simulink library "carnot"  (R2013b)
settings: Solver=ode45  StartTime=0.0  StopTime=10.0  RelTol=1e-3
undefined symbols (not defined in the file or in its folder): A, acol, Ahabit, Awin, Azimuth_Angle, AziWin, B, C, c1, c4, capc, caph, CarnotCallbacks_Density, CarnotCallbacks_Enthalpy, CarnotCallbacks_Enthalpy2Temperature, CarnotCallbacks_Entropy, CarnotCallbacks_Evaporation_Enthalpy, CarnotCallbacks_GlobalMessageLevel, CarnotCallbacks_Grashof, CarnotCallbacks_Heat_Capacity, CarnotCallbacks_Kinematic_Viscosity, CarnotCallbacks_Prandtl, CarnotCallbacks_Saturation_Property, CarnotCallbacks_Saturation_Temperature, CarnotCallbacks_Saturation_Value_Water, CarnotCallbacks_Specific_Volume, CarnotCallbacks_Thermal_Conductivity, CarnotCallbacks_Vapour_Content, CarnotCallbacks_Vapour_Pressure, con, cond, d, Dd, density, dfin, dia, DiameterLastPiece, DPConstant, dpipe, DPLinear, DPQuadratic, emission_out, fluid, FluidMix, FluidType, FPC, frame, g, GeodeticHeight, Gwin, heat_capacity, hgt, HP, Hroom, ID, inlet, K, l, lin, lpipe ... (+29)
undefined symbols (not defined in the file): c2, c3, c5, c6, cwall, dactive, height, mc, mID, rho, tau, UAneighbour, UAwall, uloss
libraries: carnot x333, simulink x25, simulink_extras x7
(part 6 of 16)

== system carnot/Load/Hot_Water_Tapping ==
  Applications : Subsystem
      mask Display: plot(0,0,100,100,[10,10,40,40,10],[10,40,40,10,10],[50,70,90,50],[30,65,30,30],[20,10,10,20,30,40,40,30,20],[50,60,70,80,80,70,60,50,50])
  DHW_Energy_Tapping : Subsystem  mask{mdot_nom=1/60, times=[7     7.1 7.5   8.083 8.25  8.5   8.75  9     9.5   10.5  11.5  11.75 12.75 14.5  15.5  16.5  18    18.25 18.5  19    20.5  21.25 21.5]*3600, energies=[0.105 1.4 0.105 0.105 0.105 0.105 0.105 0.105 0.105 0.105 0.105 0.105 0.315 0.105 0.105 0.105 0.105 0.105 0.105 0.105 0.735 0.105 1.4 ]*36e5, dT_set=[30    30  30    30    30    30    30    30    30    30    30    30    45    30    30    30    30    30    30    30    45    30    30  ], coeffs=[3     6   3     3     3     3     3     3     3     3     3     3     4     3     3     3     3     3     3     3     4     3     6   ]}
      mask prompts: mdot_nom "nominal massflow [kg/s]"; times "vector of start times of taps [s]"; energies "vector of energies of taps [J]"; dT_set "vector of delta set temperatures of taps [K]"; coeffs "vector of coefficients of nominal massflow of taps [-]"
      mask Display: disp('dhw_EN13203')
  EU_Tapping_Cycle : Subsystem  mask(European tapping cycles){eu_tap=L}
      mask prompts: eu_tap "EU Tapping Cycle Number"
      mask help: European tapping cycles according to EN 13203.
      mask init:
      | % times in h, energies in kWh, massflow in kg/min
      | % will be transformed to s, J at kg/s the end
      | switch(eu_tap)
      |     case 1  % profile 3XS   0.345 kWh
      |         times =    [7.000   7.083   7.250   7.433   7.500   9.000   9.500   11.50   11.75   12.00   12.50   12.75   14.50   15.00   15.50   16.00   18.50   19.00   19.50   21.25   21.50   21.58   21.75 ];
      |         energies = [0.015   0.015   0.015   0.015   0.015   0.015   0.015   0.015   0.015   0.015   0.015   0.015   0.015   0.015   0.015   0.015   0.015   0.015   0.015   0.015   0.015   0.015   0.015 ];
      |         dT_set =   [30      30      30      30      30      30      30      30      30      30      30      30      30      30      30      30      30      30      30      30      30      30      30  ];
      |         mdot =     [2       2       2       2       2       2       2       2       2       2       2       2       2       2       2       2       2       2       2       2       2       2       2   ];
      | 
      |     case 2  % profile XXS   2.1 kWh
      |         times =    [7.000   7.500   8.500   9.500   11.50   11.75   12.00   12.50   12.75   18.00   18.25   18.50   19.00   19.50   20.00   20.75   21.00   21.25   21.58   21.75 ];
      |         energies = [0.105   0.105   0.105   0.105   0.105   0.105   0.105   0.105   0.105   0.105   0.105   0.105   0.105   0.105   0.105   0.105   0.105   0.105   0.105   0.105 ];
      |         dT_set =   [30      30      30      30      30      30      30      30      30      30      30      30      30      30      30      30      30      30      30      30    ];
      |         mdot =     [2       2       2       2       2       2       2       2       2       2       2       2       2       2       2       2       2       2       2       2     ];
      | 
      |     case 3  % profile XS    2.1 kWh
      |         times =    [7.500   12.75   21.50   ];
      |         energies = [0.525   0.525   1.05    ];
      |         dT_set =   [30      30      30      ];
      |         mdot =     [3       3       3       ];
      |     
      |     case 4  % profile S     2.1 kWh
      |         times =    [7.000   7.500   8.500   9.500   11.50   11.75   12.75   18.00   18.25   20.50   21.50   ];
      |         energies = [0.105   0.105   0.105   0.105   0.105   0.105   0.315   0.105   0.105   0.420   0.525   ];
      |         dT_set =   [30      30      30      30      30      30      45      30      30      45      30      ];
      |         mdot =     [3       3       3       3       3       3       4       3       3       4       5       ];
      |     
      |     case 5 % Profile M      5.845 kWh
      |         times =    [7.000 7.083 7.500 8.016 8.250 8.5   8.750 9.000 9.500 10.50 11.50 11.75 12.75 14.50 15.50 16.50 18.00 18.25 18.50 19.00 20.50 21.25 21.5];
      |         energies = [0.105 1.4   0.105 0.105 0.105 0.105 0.105 0.105 0.105 0.105 0.105 0.105 0.315 0.105 0.105 0.105 0.105 0.105 0.105 0.105 0.735 0.105 1.4 ];
      |         dT_set =   [30    30    30    30    30    30    30    30    30    30    30    30    45    30    30    30    30    30    30    30    45    30    30  ];
      |         mdot   =   [3     6     3     3     3     3     3     3     3     3     3     3     4     3     3     3     3     3     3     3     4     3     6   ];
      |         
      |     case 6 % profile L      11.655 kWh
      |         times =    [7.000 7.083 7.500 7.750 8.083 8.416 8.500 8.750 9.000 9.500 10.50 11.50 11.75 12.75 14.50 15.50 16.50 18.00 18.25 18.50 19.00 20.50 21.00 21.5 ];
      |         energies = [0.105 1.4   0.105 0.105 3.605 0.105 0.105 0.105 0.105 0.105 0.105 0.105 0.105 0.315 0.105 0.105 0.105 0.105 0.105 0.105 0.105 0.735 3.605 0.105];
      |         dT_set   = [30    30    30    30    30    30    30    30    30    30    30    30    30    45    30    30    30    30    30    30    30    45    30    30   ];
      |         mdot     = [3     6     3     3     10    3     3     3     3     3     3     3     3     4     3     3     3     3     3     3     3     4     10    3    ];
      |         
      |     case 7  % profile XL      19.07 kWh
      |         times =    [7.000 7.25  7.433 7.75  8.016 8.250 8.500 8.750 9.000 9.500 10.00 10.50 11.00 11.50 11.75 12.75 14.50 15.00 15.50 16.00 16.50 17.00 18.00 18.25 18.50 19.00 20.50 20.76 21.25 21.5 ];
      |         energies = [0.105 1.82  0.105 4.42  0.105 0.105 0.105 0.105 0.105 0.105 0.105 0.105 0.105 0.105 0.105 0.735 0.105 0.105 0.105 0.105 0.105 0.105 0.105 0.105 0.105 0.105 0.735 4.420 0.105 4.42 ];
      |         dT_set   = [30    35    30    30    30    30    30    30    30    30    30    30    30    30    45    45    30    30    30    30    30    30    30    35    35    30    45    35    30    35   ];
      |         mdot     = [3     6     3     10    3     3     3     3     3     3     3     3     3     4     3     3     3     3     3     3     3     4     10    3     3     3     4     10    3     10   ];
      |         
      |     case 8  % profile XXL      24.53 kWh
      |         times =    [7.000 7.25  7.433 7.75  8.016 8.250 8.500 8.750 9.000 9.500 10.00 10.50 11.00 11.50 11.75 12.75 14.50 15.00 15.50 16.00 16.50 17.00 18.00 18.25 18.50 19.00 20.50 20.76 21.25 21.5 ];
      |         energies = [0.105 1.82  0.105 6.24  0.105 0.105 0.105 0.105 0.105 0.105 0.105 0.105 0.105 0.105 0.105 0.735 0.105 0.105 0.105 0.105 0.105 0.105 0.105 0.105 0.105 0.105 0.735 6.240 0.105 6.24 ];
      |         dT_set   = [30    35    30    35    30    30    30    30    30    30    30    35    30    45    45    45    30    30    30    30    30    30    30    35    35    30    45    35    35    35   ];
      |         mdot     = [3     6     3     10    3     3     3     3     3     3     3     3     4     3     3     4     3     3     3     3     3     3     3     3     3     3     4     16    10    16   ];
      |         
      |     case 9  % profile 3XL      46.76 kWh
      |         times =    [7.00  8.016 9.000 10.50 11.75 12.75 15.50 18.50 20.50 21.5 ];
      |         energies = [11.2  5.04  1.68  0.840 1.68  2.520 2.520 3.36  5.88  12.04];
      |         dT_set   = [35    30    30    35    30    45    30    30    45    35   ];
      |         mdot     = [48    24    24    24    24    32    24    24    32    48   ];
      |         
      |     case 10 % profile 4XL      93.52 kWh
      |         times =    [7.000 8.016 9.000 10.50 11.75 12.75 15.50 18.50 20.50 21.5 ];
      |         energies = [22.40 10.08 3.36  1.680 3.360 5.04  5.04  6.72  11.76 24.08];
      |         dT_set   = [35    30    30    30    30    45    30    30    45    35   ];
      |         mdot     = [96    48    48    10    48    64    48    48    64    96   ];
      |         
      |     otherwise
      |         disp('Wrong definition of tapping profile')
      | end
      | energies = energies*36e5;
      | times = times*3600;
      | mdot = mdot/60;
      mask TypeOptions eu_tap: 3XS | XXS | XS | S | M | L | XL | XXL | 3XL | 4XL
      mask Display: disp('EU tapping\n from 3XS\nto 4XL')
  T_cold_Water_Location : Subsystem  mask(water tap){loc=Wuerzburg}
      mask prompts: loc "Location"
      mask help:
      | The block models a tap, that produces a constant massflow of a fluid at given times.
      | control = 1 is full massflow, control = 0 is no massflow.
      | The temperature is a sine wave according to:
      |
      | T(out) = T(mean) + T(amplitude) * sin( 2*PI*(SimulationDay + DayPhaseShift) / 365 )
      mask init:
      | switch loc
      |     case 1  % Athens
      |         T = 15;
      |         Tamp = 5;
      |         dshift = -20;
      |         disp('check temperatures for Athens')
      |     case 2  % Barcelona
      |     case 4  % Madrid
      |         T = 13.5;
      |         Tamp = 4.5;
      |         dshift = -19;
      |     case 3  % Lyon
      |         T = 12;
      |         Tamp = 4;
      |         dshift = -80;
      |         disp('check temperatures for Lyon')
      |     case 5  % Stockholm
      |         T = 8.5;
      |         Tamp = 6.4;
      |         dshift = -80;
      |         disp('check temperatures for Stockholm')
      |     case 6  % Wuerzburg
      |         T = 10;
      |         Tamp = 3;
      |         dshift = -137;
      |     case 7  % Zuerich        
      |         T = 9.7;
      |         Tamp = 6.3;
      |         dshift = -60;
      |         disp('check temperatures for Zuerich')
      |     otherwise
      |         T = 10;
      |         Tamp = 3;
      |         dshift = -137;
      | end
      mask Help: eval('man (''water_tap'')')
      mask TypeOptions loc: Athens | Barcelona | Lyon | Madrid | Stockholm | Wuerzburg | Zuerich
      mask Display:
      | str = ['Athens   ';'Barcelona';'Lyon     ';'Madrid   ';'Stockholm';'Wuerzburg';'Zuerich  '];
      | disp(str(loc,:))
  T_cold_Water_Season : Subsystem  mask(water tap){form=sine wave, month1=February, temp1=6, month2=August, temp2=14}
      mask prompts: form "temperature distribution"; month1 "month with min. temp"; temp1 "minimal temperature [°C]"; month2 "month with max. temp"; temp2 "maximal temperature [°C]"
      mask help:
      | The block models a tap, that produces a constant massflow of a fluid at given times.
      | control = 1 is full massflow, control = 0 is no massflow.
      | The temperature of the water varies during the year.
      mask Help: eval('man (''water_tap'')')
      mask TypeOptions form: sine wave | linear
      mask TypeOptions month1: January | February | March | April | May | June | July | August | September | October | November | December
      mask TypeOptions month2: January | February | March | April | May | June | July | August | September | October | November | December
      mask Display: plot(0,-10,115,110,[0,0],[100,0],[100,0],[50,50],[100,70,20,0],[44,70,30,44])
  T_cold_Water_Sine : Subsystem  mask(water tap){T=10, Tamp=3, dshift=-137}
      mask prompts: T "mean temperature [degree centigrade]"; Tamp "amplitude of the sine [k]"; dshift "phase shift of the sine in [days]"
      mask help:
      | The block models a tap, that produces a constant massflow of a fluid at given times.
      | control = 1 is full massflow, control = 0 is no massflow.
      | The temperature is a sine wave according to:
      |
      | T(out) = T(mean) + T(amplitude) * sin( 2*PI*(SimulationDay + DayPhaseShift) / 365 )
      mask Help: eval('man (''water_tap'')')
      mask Display: plot(0,-10,115,110,[0,0],[100,0],[100,0],[50,50],[100,90,80,70,60,50,40,30,20,10,0],[50,38,30,30,38,50,61,69,69,61,50])
  Water_Tap : Subsystem  mask(water tap){dia=0.02, p=2e5}
      mask prompts: dia "diameter at outlet [m]"; p "system pressure [Pa]"
      mask help:
      | The block models a tap, that produces a constant massflow of a fluid at given times.
      | control = 1 is full massflow, control = 0 is no massflow.
      mask init:
      | fluid = 1; %water
      | mix = 0;
      | dia = max(0.001, dia);
      | p = max(p, 0);
      mask Help: eval('man (''water_tap'')')
      mask Display: plot(-10,10,90,90,[44,67,67,45,45,40,40,44],[80,80,72,72,60,60,76,80],[60,45],[90,90],[53,53],[80,90],[24,29,70,75,24],[30,10,10,30,30],[42,42],[32,58],[46,44],[34,54],[38,40],[34,56])
  create_mdot : Subsystem  mask(Create Massflow Profile){}
      settings: OpenFcn=CarnotCallbacks_create_mdot('initialize',gcb);
      mask Help: web(fullfile(path_carnot('help'),'create_mdot.html'),'-helpbrowser')
  mdot_40_20_40 : Subsystem  mask(Repeating Tapping Profile){period=24*3600, rep_seq_t=[7 12 19]*3600, rep_seq_d=[0.2 0.1 0.2]*3600, rep_seq_y=[1 1 1]*200/1800}
      mask prompts: period "Time period in s"; rep_seq_t "Time values in s"; rep_seq_d "Duration in s"; rep_seq_y "Output values:"
      mask help:
      | Period must be larger than the last time value.
      | Time values must be monotonically ingreasing. Give one time value for the start of the tapping.
      | Duration is a vector with the same number of elements than the time values. Each duration corresponts to one time value.
      | The number of output values must be the same as the number of time values. Each output value corresponds to one time value.
      mask init: same as carnot/Load/General/Repeating_Profile
      mask Help:
      | Period must be larger than the last time value.
      | Time values must be monotonically ingreasing. Give one time value for the start of the tapping.
      | Duration is a vector with the same number of elements than the time values. Each duration corresponts to one time value.
      | The number of output values must be the same as the number of time values. Each output value corresponds to one time value.
      mask Display: plot( disp_t, disp_y )
  mdot_DHWcalc : Subsystem  mask(dhw from file){file=DHW0001_DHW, ext=.txt, dt=60}
      mask prompts: file "Name of file"; ext "Extension of file"; dt "Time step duration [s]"
      mask help:
      | Input for files created with the dhw-calc software.
      | These files contain only the massflow in kg/h, the conversion to kg/s is done in the block.
      | Details and manual at
      | http://solar.umwelt-uni-kassel.de/downloads.de.html
      mask init:
      | eval(['load(''' file ext ''');']);
      | eval([file ' = [ [0:dt:(length(' file ')-1)*dt]'' ' file '];' ]);
      | set_param([gcb '/dhw_from_Workspace'], 'VariableName', file);
      mask Help: eval('man (''dhw_from_file'')')
      mask TypeOptions ext: .dat | .txt
      mask Display: disp(file)

== system carnot/Load/Houses ==
  Room_Floor_Heating : Subsystem  mask(room){t0=20, temp_neighbour=20}
      mask prompts: t0 "start temperature of rooms in °C"; temp_neighbour "temperature of rooms above and below in °C"
      mask help:
      | The block models of a heat transfer characteristic of two neighbour rooms.
      | Use "look under mask" to set up the models parameters (initial conditions,
      | floors and wall characteristics...)
      mask init:
      | AIV_neighbour = [0 temp_neighbour temp_neighbour 0 0 0 0 0 0];
      | zonefloordist2grnd = 0;
      mask Help: web(fullfile(path_carnot('help'),'Room_Floor_Heating.html'),'-helpbrowser')
      mask Display: plot(0,0,100,100,[30,30,60,60,30],[20,50,50,20,20],[47,47,56,56,47],[40,30,30,40,40],[42,42,34,34],[20,40,40,20],[62,45,28],[48,70,48])
  Room_Radiator : Subsystem  mask(room){t0=20, temp_neighbour=20}
      mask prompts: t0 "start temperature of rooms in °C"; temp_neighbour "temperature of rooms above and below in °C"
      mask help:
      | The block models of a heat transfer characteristic of two neighbour rooms.
      | Use "look under mask" to set up the models parameters (initial conditions,
      | floors and wall characteristics...)
      mask init:
      | AIV_neighbour = [0 temp_neighbour temp_neighbour 0 0 0 0 0 0];
      | zonefloordist2grnd = 0;
      mask Help: web(fullfile(path_carnot('help'),'Room_Radiator.html'),'-helpbrowser')
      mask Display: plot(0,0,100,100,[30,30,60,60,30],[20,50,50,20,20],[47,47,56,56,47],[40,30,30,40,40],[42,42,34,34],[20,40,40,20],[62,45,28],[48,70,48])
  Simple_House : Subsystem  mask(simple house){Ahabit=30, Hroom=2.5, Floorsize=[5 6], UAwall=0.162*(30)+0.182*((5+6)*2*2.5 -(4+0+0+0)), UAneighbour=0, Uground=0  %0.18 wenn Wert verlangt, mc=0.5e6*30   % 0.5 MJ/m2/K, shade=0.75, tini=20, Awin=[4 0 0 0], AziWin=[0 90 -180 -90], Uwin=[1    1   1    1]*1.5, Gwin=[1    1   1    1]*0.7*(1-0.15), vent=0.4, rec=0, heatload=2000, dpcoeff=[10 100], delta_t_nom=50, n_rad=1.1, mass_times_cap=40e6}
      mask prompts: Ahabit "Living surface in m²"; Hroom "height of rooms in m"; Floorsize "Dimensions of slab in m [length width]"; UAwall "Total heat transfer to ambient (walls/roof) in W/K"; UAneighbour "Total heat transfer to neighbour inW/K"; Uground "Heat transfer coeffient to ground in W/m²/K"; mc "Total thermal capacity in J/K"; shade "Shading factor [0..1] when T room > 4 K + T_init"; tini "Initial temperature"; Awin "Surface of 4 windows in m² (vector)"; AziWin "Orientation of 4 windows (south 0, east -90,west 90)"; Uwin "Heat loss coefficient 4 windows in W/m²/K [vector]"; Gwin "Light transmittance 4 windows (0..1) * (1 - frame_part) [vector]"; vent "Ventilation rate in 1/h"; rec "Heat recovery (0..1)"; heatload "Heating capacity radiator  [W]"; dpcoeff "Pressure drop coefficients [linear quadratic] in Pa/(kg/s), Pa/(kg/s)²"; delta_t_nom "Nominal delta T (average radiator temperature - room temperature) [K]"; n_rad "Radiator exponent"; mass_times_cap "Mass*capacity of heating system [J/K]"
      mask help:
      | Simple model of 1-node room or house. The differential equation
      | (m*c)house * dT/dt = solar_gain + internal_gain + heating_power - losses_to_ambient - losses_to_neighbour_room
      | is solved.
      | The heating power is generated by a radiator or floor heating system.
      | The windows have an automatic shading (shading factor) if room temperature rises 4 K above initial temperature.
      | solar gain = Solar_Radiation_on_window * light_transmittance * shading_factor
      | Use "look under mask" to set up the models parameters (initial conditions, surfaces characteristics...).
      | A usual value for the internal gains is 2.3 W/m².
      mask init:
      | invmc = 1/mc;
      | rec = max(0,min(1,rec));
      | Gwin = max(0,min(1,Gwin));
      | shade = max(0, min(1, shade));
      mask Help: web(fullfile(path_carnot('help'),'simple_house.html'),'-helpbrowser')
      mask Display: plot(0,-15,80,100,[30,30,60,60,30],[20,50,50,20,20],[47,47,56,56,47],[40,30,30,40,40],[42,42,34,34],[20,40,40,20],[62,45,28],[48,70,48])
  Simple_House_ISO_GroundModel : Subsystem  mask(Simple House with ISO 13370 Ground Model){Ahabit=140, Hroom=2.6, Floorsize=[7 10], UAwall=0.162*(54.6+26.4)+0.182*((45.7+56.0)*2 -(12+4+3+4)), UAneighbour=0, Uground=0.1, mc=0.5e6*140 % 0.5 MJ/m2/K, shade=0.75, tini=20, Awin=[12 4 3 4], AziWin=[0 90 -180 -90], Uwin=[1    1   1    1]*1.0, Gwin=[1    1   1    1]*0.585*(1-0.15), vent=0.4, rec=0.6, heatload=1792, delta_t_nom=15, n_rad=1.1, mass_times_cap=40e6, dpcoeff=[10 100]}
      mask prompts: Ahabit "Living surface in m²"; Hroom "height of rooms in m"; Floorsize "Dimensions of slab in m [length width]"; UAwall "Total heat transfer to ambient (walls/roof) in W/K"; UAneighbour "Total heat transfer to neighbour inW/K"; Uground "Heat transfer coeffient of slab to ground in W/m²/K"; mc "Total thermal capacity in J/K"; shade "Shading factor [0..1] when T room > 4 K + T_init"; tini "Initial temperature"; Awin "Surface of 4 windows in m² (vector)"; AziWin "Orientation of 4 windows (south 0, east -90,west 90)"; Uwin "Heat loss coefficient 4 windows in W/m²/K [vector]"; Gwin "Light transmittance 4 windows (0..1) * (1 - frame_part) [vector]"; vent "Ventilation rate in 1/h"; rec "Heat recovery (0..1)"; heatload "Heating capacity radiator  [W]"; delta_t_nom "Nominal delta T (average radiator temperature - room temperature) [K]"; n_rad "Radiator exponent"; mass_times_cap "Mass*capacity of heating system [J/K]"; dpcoeff "Pressure drop coefficients [linear quadratic] in Pa/(kg/s), Pa/(kg/s)²"
      mask help:
      | Uses the simple model of 1-node room or house. The heating power is generated by a radiator or floor heating system.
      | The windows have an automatic shading (shading factor) if room temperature rises 4 K above initial temperature.
      | solar gain = Solar_Radiation_on_window * light_transmittance * shading_factor
      | The ground model of ISO 13370 is used to calculate the losses to the ground. Remember to set the values of the model according to the set point of the room temperature and the weather data.
      mask init:
      | invmc = 1/mc;
      | rec = max(0,min(1,rec));
      | Gwin = max(0,min(1,Gwin));
      | shade = max(0, min(1, shade));
      mask Help: web(fullfile(path_carnot('help'),'simple_house.html'),'-helpbrowser')
      mask Display:
      | plot(-20,-30,120,100,[10,10,90,90,10],[0,50,50,0,0],...
      |     [100,60,40,0],[40,80,80,40],[20,34,34,20,20],[40,40,20,20,40],...
      |     [60,60,40,40],[0,40,40,0],[65,80,80,65,65],[40,40,20,20,40],...
      |     [47,54,54,47,47],[35,35,4,4,35],[45,41],[20,20])
  Simple_House_ISOgm_CONF : Subsystem  mask(Simple House with ISO 13370 Ground Model){parameterfile=Default_SimpleHouseISOgm, tini=20}
      mask prompts: parameterfile "Parameter set"; tini "Initial temperature in °C"
      mask help: Preconfigurated parameter sets.
      mask init:
      | % path definitions
      | intpath = fullfile(path_carnot('intlibsl'), ...
      |     'Load','Houses','Simple_House_ISOgm_CONF','parameter_set');
      | pubpath = fullfile(path_carnot('libsl'), ...
      |     'Load','Houses','Simple_House_ISOgm_CONF','parameter_set');
      | 
      | [namelist, lib] = CarnotCallbacks_getConfNamelist(intpath,pubpath);
      | 
      | if ~lib
      |     myMaskStylesVar{1} = ['popup(', namelist,')'];
      |     myMaskStylesVar{2} = 'edit';
      |     set_param(gcb, 'MaskStyles', myMaskStylesVar)
      | end
      | 
      | if exist(fullfile(intpath,[parameterfile '.mat']))
      |     load(fullfile(intpath,parameterfile));
      | else
      |     load(fullfile(pubpath,parameterfile));
      | end
      mask Help: web(fullfile(path_carnot('help'),'simple_house.html'),'-helpbrowser')
      mask TypeOptions parameterfile: Default_SimpleHouseISOgm
      mask Display:
      | % user defined picture file
      | picfile = fullfile(path_carnot('intlibsl'), ...
      |         'Load','Houses','Simple_House_ISOgm_CONF','parameter_set', ...
      |         'Simple_House_ISOgm_CONF.jpg');
      | 
      | % show internal picture if defined
      | if ~BlockIsInCarnotLibrary ...      % if not located in library any more
      |         && exist(picfile,'file')    % AND picfile is present
      |     image(imread(picfile), [0.15 0.1 0.7 0.8])
      |     set_param(gcb, 'BackgroundColor', 'White')
      | else
      |     % show public picture
      |     plot([10,10,90,90,10]/100,[0,50,50,0,0]/100,...
      |          [100,60,40,0]/100,[40,80,80,40]/100,...
      |          [20,34,34,20,20]/100,[40,40,20,20,40]/100,...
      |          [60,60,40,40]/100,[0,40,40,0]/100,...
      |          [65,80,80,65,65]/100,[40,40,20,20,40]/100,...
      |          [47,54,54,47,47]/100,[35,35,4,4,35]/100,...
      |          [45,41]/100,[20,20]/100)
      |     set_param(gcb, 'BackgroundColor', 'Orange')
      | end
      | 
      | % port labels
      | port_label('input',1,'WDB')
      | port_label('input',2,'THB')
      | port_label('output',1,'Hdat')
      | port_label('output',2,'THB')
  heat_transfer : Subsystem
      mask Display: plot(0,0,100,100,[10,10,40,40,10],[10,40,40,10,10],[50,70,90,50],[30,65,30,30],[20,10,10,20,30,40,40,30,20],[50,60,70,80,80,70,60,50,50])
  room_nodes : Subsystem
      mask Display: plot(0,0,100,100,[10,10,40,40,10],[10,40,40,10,10],[50,70,90,50],[30,65,30,30],[20,10,10,20,30,40,40,30,20],[50,60,70,80,80,70,60,50,50])
  ventilation_heating : Subsystem
      mask Display: plot(0,0,100,100,[10,10,40,40,10],[10,40,40,10,10],[50,70,90,50],[30,65,30,30],[20,10,10,20,30,40,40,30,20],[50,60,70,80,80,70,60,50,50])
  wall_floor : Subsystem
      mask Display: plot(0,0,100,100,[10,10,40,40,10],[10,40,40,10,10],[50,70,90,50],[30,65,30,30],[20,10,10,20,30,40,40,30,20],[50,60,70,80,80,70,60,50,50])

== system carnot/New_Blocks/ReadFile ==
  S-Function : S-Function  FunctionName=readfile  Parameters=number timedep filename  EnableBusSupport=off
  dummy constant : Constant  Value=0
  data : Outport
  wires:
  dummy constant/1 -> S-Function/1
  S-Function/1 -> data/1

== system carnot/New_Blocks/ground_storage_U_tube ==
  WDB : Inport
  THBin : Inport  Port=2
  Tsurface : Inport  Port=3
  Tbottom : Inport  Port=4
  Demux : Demux  Outputs=[3*mpts 1 1 3]
  Demux1 : Demux  Outputs=[1 1 1 1 2 1 3]
  Demux2 : Demux  Outputs=[10 10]
  Matrix Gain : Gain  Gain=[1-1/zn:-1/zn:0]'  SaturateOnIntegerOverflow=on  OutDataTypeStr=Inherit: Same as input  ParamDataTypeStr=Inherit: Same as input
  Mux : Mux  Inputs=10
  Mux1 : Mux  Inputs=8
  Open_Surface : carnot/Storage/Thermal/surface_models/Open_Surface  albedo=0.6
  S-Function : S-Function  FunctionName=ut_stor2  Parameters=ds, hs, ce, le, dp, dh, hh, ch, lh, kp, t0, rn, zn, mpts  EnableBusSupport=off
  Sum : Sum  Inputs=+-  SaturateOnIntegerOverflow=on  InputSameDT=on  OutDataTypeStr=Inherit: Same as first input
  Sum1 : Sum  SaturateOnIntegerOverflow=on  InputSameDT=on  OutDataTypeStr=Inherit: Same as first input
  THB2THV : carnot/Toolbox/THB2THV
  THV2THB : carnot/Toolbox/THV2THB
  diameter : Constant  Value=dp
  THB : Outport
  Tnodes : Outport  Port=2
  wires:
  Mux1/1 -> THV2THB/1
  Demux/1 -> Tnodes/1
  Demux/4 -> Mux1/7  "clq"
  Demux1/7 -> Mux/8  "clq"
  Sum1/1 -> Mux/9
  Demux/2 -> Mux1/2  "Tout"
  Demux/3 -> Mux1/4  "p_out"
  S-Function/1 -> Demux/1
  WDB/1 -> Open_Surface/1
  diameter/1 -> Mux1/6
  Demux2/2 -> Mux1/8
  THBin/1 -> THB2THV/1
  Demux2/1 -> Demux1/1
  Open_Surface/1 -> Mux/1
  Demux1/1 -> Mux/2, Mux1/1  "ID"
  Mux/1 -> S-Function/1
  Demux1/2 -> Mux/3  "T"
  Demux1/4 -> Mux/5  "p"
  Demux1/6 -> Mux/7  "d"
  Demux1/3 -> Mux/4, Mux1/3  "mdot"
  Demux1/5 -> Mux/6, Mux1/5  "fluid, mix"
  Tsurface/1 -> Sum/1
  Sum/1 -> Matrix Gain/1
  Matrix Gain/1 -> Sum1/1
  Tbottom/1 -> Sum/2, Mux/10, Sum1/2
  THB2THV/1 -> Demux2/1
  THV2THB/1 -> THB/1

== system carnot/Outputs/AIV_selector ==
  "[AIV]" : Inport
  Selector : Selector  InputPortWidth=9  IndexOptions=Index vector (dialog)  Indices=v  OutputSizes=1
  "[AIV]s" : Outport
  wires:
  Selector/1 -> "[AIV]s"/1
  "[AIV]"/1 -> Selector/1

== system carnot/Outputs/Display_THB1 ==
  THB_yellow : Inport
  Selector : Selector  InputPortWidth=20  IndexOptions=Index vector (dialog)  Indices=[v]  OutputSizes=1
  THB2THV : carnot/Toolbox/THB2THV
  to_scope : Outport
  wires:
  Selector/1 -> to_scope/1
  THB_yellow/1 -> THB2THV/1
  THB2THV/1 -> Selector/1

== system carnot/Outputs/Display_THB2 ==
  THB_yellow : Inport
  THB_magenta : Inport  Port=2
  Mux : Mux  Inputs=2
  Selector : Selector  InputPortWidth=20  IndexOptions=Index vector (dialog)  Indices=[v]  OutputSizes=1
  Selector1 : Selector  InputPortWidth=20  IndexOptions=Index vector (dialog)  Indices=[v]  OutputSizes=1
  THB2THV1 : carnot/Toolbox/THB2THV
  THB2THV2 : carnot/Toolbox/THB2THV
  to_scope : Outport
  wires:
  THB_yellow/1 -> THB2THV1/1
  Selector/1 -> Mux/1
  THB_magenta/1 -> THB2THV2/1
  Mux/1 -> to_scope/1
  Selector1/1 -> Mux/2
  THB2THV1/1 -> Selector/1
  THB2THV2/1 -> Selector1/1

== system carnot/Outputs/Display_THB3 ==
  THB_yellow : Inport
  THB_magenta : Inport  Port=2
  THB_cyan : Inport  Port=3
  Mux : Mux  Inputs=3
  Selector : Selector  InputPortWidth=20  IndexOptions=Index vector (dialog)  Indices=[v]  OutputSizes=1
  Selector1 : Selector  InputPortWidth=20  IndexOptions=Index vector (dialog)  Indices=[v]  OutputSizes=1
  Selector2 : Selector  InputPortWidth=20  IndexOptions=Index vector (dialog)  Indices=[v]  OutputSizes=1
  THB2THV1 : carnot/Toolbox/THB2THV
  THB2THV2 : carnot/Toolbox/THB2THV
  THB2THV3 : carnot/Toolbox/THB2THV
  to_scope : Outport
  wires:
  THB2THV3/1 -> Selector2/1
  THB2THV2/1 -> Selector1/1
  THB2THV1/1 -> Selector/1
  THB_yellow/1 -> THB2THV1/1
  Selector/1 -> Mux/1
  THB_magenta/1 -> THB2THV2/1
  Mux/1 -> to_scope/1
  Selector1/1 -> Mux/2
  THB_cyan/1 -> THB2THV3/1
  Selector2/1 -> Mux/3

== system carnot/Outputs/Display_THB4 ==
  THB_yellow : Inport
  THB_magenta : Inport  Port=2
  THB_cyan : Inport  Port=3
  THB_red : Inport  Port=4
  Mux : Mux
  Selector{,1..3} (4 alike) : Selector  InputPortWidth=20  IndexOptions=Index vector (dialog)  Indices=[v]  OutputSizes=1
  THB2THV{1..4} (4 alike) : carnot/Toolbox/THB2THV
  to_scope : Outport
  wires:
  Selector3/1 -> Mux/4
  THB_red/1 -> THB2THV4/1
  Selector2/1 -> Mux/3
  THB_cyan/1 -> THB2THV3/1
  Selector1/1 -> Mux/2
  Mux/1 -> to_scope/1
  THB_magenta/1 -> THB2THV2/1
  Selector/1 -> Mux/1
  THB_yellow/1 -> THB2THV1/1
  THB2THV1/1 -> Selector/1
  THB2THV2/1 -> Selector1/1
  THB2THV3/1 -> Selector2/1
  THB2THV4/1 -> Selector3/1

== system carnot/Outputs/Display_THB5 ==
  THB_yellow : Inport
  THB_magenta : Inport  Port=2
  THB_cyan : Inport  Port=3
  THB_red : Inport  Port=4
  THB_green : Inport  Port=5
  Mux : Mux  Inputs=5
  Selector{,1..4} (5 alike) : Selector  InputPortWidth=20  IndexOptions=Index vector (dialog)  Indices=[v]  OutputSizes=1
  THB2THV{1..5} (5 alike) : carnot/Toolbox/THB2THV
  to_scope : Outport
  wires:
  THB2THV5/1 -> Selector4/1
  THB2THV4/1 -> Selector3/1
  THB2THV3/1 -> Selector2/1
  THB2THV2/1 -> Selector1/1
  THB2THV1/1 -> Selector/1
  Mux/1 -> to_scope/1
  Selector/1 -> Mux/1
  THB_yellow/1 -> THB2THV1/1
  Selector1/1 -> Mux/2
  THB_magenta/1 -> THB2THV2/1
  Selector3/1 -> Mux/4
  THB_red/1 -> THB2THV4/1
  Selector2/1 -> Mux/3
  THB_cyan/1 -> THB2THV3/1
  THB_green/1 -> THB2THV5/1
  Selector4/1 -> Mux/5

== system carnot/Outputs/Display_THB6 ==
  THB_yellow : Inport
  THB_magenta : Inport  Port=2
  THB_cyan : Inport  Port=3
  THB_red : Inport  Port=4
  THB_green : Inport  Port=5
  THB_blue : Inport  Port=6
  Mux : Mux  Inputs=6
  Selector{,1..5} (6 alike) : Selector  InputPortWidth=20  IndexOptions=Index vector (dialog)  Indices=[v]  OutputSizes=1
  THB2THV{1..6} (6 alike) : carnot/Toolbox/THB2THV
  to_scope : Outport
  wires:
  THB_blue/1 -> THB2THV6/1
  Selector5/1 -> Mux/6
  Selector4/1 -> Mux/5
  THB_green/1 -> THB2THV5/1
  THB_cyan/1 -> THB2THV3/1
  Selector2/1 -> Mux/3
  THB_red/1 -> THB2THV4/1
  Selector3/1 -> Mux/4
  THB_magenta/1 -> THB2THV2/1
  Selector1/1 -> Mux/2
  THB_yellow/1 -> THB2THV1/1
  Selector/1 -> Mux/1
  Mux/1 -> to_scope/1
  THB2THV1/1 -> Selector/1
  THB2THV2/1 -> Selector1/1
  THB2THV3/1 -> Selector2/1
  THB2THV4/1 -> Selector3/1
  THB2THV5/1 -> Selector4/1
  THB2THV6/1 -> Selector5/1

== system carnot/Outputs/S_selector ==
  "[S]" : Inport
  Selector : Selector  InputPortWidth=13  IndexOptions=Index vector (dialog)  Indices=v  OutputSizes=1
  "[S]s" : Outport
  wires:
  "[S]"/1 -> Selector/1
  Selector/1 -> "[S]s"/1

== system carnot/Outputs/Sensitive_Room_Temperature ==
  note: Sensitive temperature
  "[AIV]" : Inport
  1-share_c : Gain  Gain=1-share_c  SaturateOnIntegerOverflow=on  OutDataTypeStr=Inherit: Same as input  ParamDataTypeStr=Inherit: Same as input
  Demux : Demux  Outputs=[1 1 1 6]
  Sum : Sum  SaturateOnIntegerOverflow=on  InputSameDT=on  OutDataTypeStr=Inherit: Same as first input
  Terminator1 : Terminator
  Terminator2 : Terminator
  share_c : Gain  Gain=share_c  SaturateOnIntegerOverflow=on  OutDataTypeStr=Inherit: Same as input  ParamDataTypeStr=Inherit: Same as input
  Ts : Outport
  wires:
  Demux/1 -> Terminator2/1
  Sum/1 -> Ts/1
  1-share_c/1 -> Sum/2  "Tr"
  share_c/1 -> Sum/1  "Tc"
  Demux/4 -> Terminator1/1
  "[AIV]"/1 -> Demux/1
  Demux/2 -> share_c/1
  Demux/3 -> 1-share_c/1

== system carnot/Outputs/THV_select ==
  THV : Inport
  Selector : Selector  InputPortWidth=20  IndexOptions=Index vector (dialog)  Indices=[v]  OutputSizes=1
  out : Outport  InitialOutput=0
  wires:
  Selector/1 -> out/1
  THV/1 -> Selector/1

== system carnot/Outputs/display_weather ==
  weather : Inport
  select_weather : carnot/Weather/Select_Weather  v=v
  to scope : Outport
  wires:
  select_weather/1 -> to scope/1
  weather/1 -> select_weather/1

== system carnot/Source/Boiler ==
  Condensing_Boiler : Subsystem  mask(Condensing Boiler){Pnom=20e3, U=3, vol=0.02, electricPower=[20 120], relativeQdot=[0.25 1], whichTforEfficiency=mean of inlet and outlet temperature, temperatures=[40  70], efficiency=[1.05 0.95; 1.0 0.9], lin=10, qua=100, Tini=20, nodes=1}
      mask prompts: Pnom "nominal power [W]"; U "heat loss coefficient [W/K]"; vol "volume of the boiler [m³]"; electricPower "Electric power in W (vector, index from relative power)"; relativeQdot "relative power in 0..1 (vector for row index)"; whichTforEfficiency "Efficiency table based on"; temperatures "Temperature in °C  (vector for column index)"; efficiency "Efficiency data in 0..1 (matrix)"; lin "pressure drop linear in massflow [Pa*s/kg]"; qua "pressure drop quadratic in massflow [Pa*s²/kg²]"; Tini "initial temperature [degree centigrade]"; nodes "number of nodes"
      mask help: Multinode one-dimensional model of a boiler. Condensing effects are taken in account by an efficiency lookup table.
      mask Help: web(fullfile(path_carnot('help'),'Condensing_Boiler.html'),'-helpbrowser')
      mask TypeOptions whichTforEfficiency: mean of inlet and outlet temperature | inlet temperature | outlet temperature
      mask Display:
      | plot(-20,0,120,100,[10,90,90,10,10],[10,10,20,20,10],[80,80,20,20],[20,90,90,20],[20,70,70,20],[24,24,30,30],[32,30,28],[30,40,30],[43,40,38],[30,40,30],[53,50,47],[30,40,30],[63,60,57],[30,40,30],[35,32,30,29,31,36,39,40,37,35],[75,69,65,58,50,49,53,59,68,75],[57,54,51,51,53,58,62,62,59,57],[76,71,67,58,49,48,54,60,69,76])
      | port_label('input',1,'Ta')
      | port_label('input',2,'THB')
      | port_label('input',3,'ctr')
      | port_label('input',4,'fuel')
      | port_label('output',1,'THB')
      | port_label('output',2,'Bdat')
  Condensing_Boiler_CONF : Subsystem  mask(Configurated Condensing Boiler){parameterfile=DefaultCondensingBoiler, tini=20}
      mask prompts: parameterfile "Parameter set"; tini "Inital temperature in °C"
      mask help:
      | Multinode one-dimensional model of a boiler. Condensing effects are taken in account by an efficiency lookup table.
      | This block uses predefined parameter sets.
      mask init:
      | B = CarnotCallbacks_CondensingBoilerConf(parameterfile);
      | relQdotMin = B.QdotMin/B.Qdotnom;
      mask Help: web(fullfile(path_carnot('help'),'Condensing_Boiler_CONF.html'),'-helpbrowser')
      mask TypeOptions parameterfile: DefaultCondensingBoiler | Vitodens_200_13kW | Vitodens_200_19kW | Vitodens_200_26kW | Vitodens_200_35kW
      mask Display:
      | % user defined picture file
      | picfile = fullfile(path_carnot('intlibsl'), ...
      |         'Source','Boiler','Condensing_Boiler_CONF','parameter_set', ...
      |         'Condensing_Boiler_CONF.jpg');
      | 
      | % show public picture
      | plot(0,0,1,1,[10,90,90,10,10]/100,[10,10,20,20,10]/100,[80,80,20,20]/100, ...
      |     [20,90,90,20]/100,[20,70,70,20]/100,[24,24,30,30]/100,[32,30,28]/100, ...
      |     [30,40,30]/100,[43,40,38]/100,[30,40,30]/100,[53,50,47]/100, ...
      |     [30,40,30]/100,[63,60,57]/100,[30,40,30]/100, ...
      |     [35,32,30,29,31,36,39,40,37,35]/100,[75,69,65,58,50,49,53,59,68,75]/100, ...
      |     [57,54,51,51,53,58,62,62,59,57]/100,[76,71,67,58,49,48,54,60,69,76]/100)
      | 
      | % show internal picture if defined
      | if ~BlockIsInCarnotLibrary    % if not located in library any more
      |     if exist(picfile,'file')
      |         image(imread(picfile), [0.2, 0, 0.6, 1])
      |         disp('4')
      |         set_param(gcb, 'BackgroundColor', 'White')
      |         disp('5')
      |     end
      | end
      | % port labels
      | port_label('input',1,'Ta')
      | port_label('input',2,'THB')
      | port_label('input',3,'ctr')
      | port_label('input',4,'fuel')
      | port_label('output',1,'THB')
      | port_label('output',2,'Bdat')
  Electric_Heater : Subsystem  mask(Electric Heater){}
      mask help: Heats the mass flow defined by the thermo-hydraulic bus with an electric power [W] entering the block.
      mask Help: web(fullfile(path_carnot('help'),'electric_heating.html'),'-helpbrowser')
      mask Display:
      | plot(0,0,100,100,[50,50,60,40,50],[55,40,70,60,90],[59,50],[48,40])
      | port_label('input',1,'THB')
      | port_label('input',2,'Qdot')
      | port_label('output',1,'THB')

== system carnot/Source/Chiller ==
  Absorption_Chiller_ddT : Subsystem  mask(Absorption chiller model){E=1.2, sE=0.42, rE=0.9, sG=0.51, rG=2/0.51, dpe=[100 1e4], dpg=[100 1e4], Pel_p=80}
      mask prompts: E "E (A = 1+E)"; sE "s_e"; rE "r_e"; sG "s_g"; rG "r_g"; dpe "[linear quadratic] massflow dependant pressure drop evaporator in [Pa]"; dpg "[linear quadratic] massflow dependant pressure drop generator in [Pa]"; Pel_p "Pel solution pump [W]"
      mask help:
      | Empirical model of an absorption chiller based on the fitted deltadelta_t'
      | model from A. Kühn (2005) :
      |
      | Linear model:
      |  deltadelta_t'=t_G - A*t_AC + E*t_E
      |  Qdot_E = s_e * deltadelta_t' + r_e
      |  Qdot_G = s_g * deltadelta_t' + r_g
      |
      | Use acm_param.m to determine A, E, s_e, r_e, s_g and r_g with
      | characterisitics of the absorption chiller.
      mask Display: disp('Absorption\nChiller\nDeltaDeltaT\nModel')
  Compression_Air_Water_Chiller : Subsystem  mask(compression air/water chiller){Q_Nom=15}
      mask prompts: Q_Nom "Q_Nom [kW]"
      mask help:
      | This block is based on the characteristic curves for cooling capacity and
      | coefficient of performance of the reversible air-to-water heat pump with waste heat recovery LI 16TER+ by Dimplex.
      | The cooling capacity, coefficient of performance, electrical power and THV_WATER_OUT are calculated.
      | The air THV is not calculated due to missing interest.
      | The scaling is based on the point of 11.9 kW.
      |
      | Enter the cooling capacity for the point
      | T_AIR_IN= 30°C, T_WATER_OUT= 7°C.
      | A capacity between 5..50 kW is recommended.
      mask Help: web(fullfile(path_carnot('help'),'compression_chiller.html'),'-helpbrowser')
  Cooling_Tower : Subsystem  mask(Closed Circuit Cooling Tower){}
      mask help:
      | performance data
      | wet-bulb temperature - 15°C ... 24°C
      | rpm fan - 248 1/min (30%) ... 824 1/min (100%)
      | fluid temperature - 26°C ... 44°C
      | fluid flow rate - 1,07 l/s ... 3,03 l/s
      | water/glykol - 0 % ... 100%
      |
      | data logging:
      | wet-bulb temperature....[°C]   (ambient air)
      | rpm fan.........................[%]
      | v_dot fan......................[m³/s]
      | rpm fan.........................[1/min]
      | rel_hum.........................[%]     (ambient air)
      | t_air..............................[°C]    (ambient air)
      | energy ct......................[kJ]    (fan motor + recirculating spray pump)
      | power ct.......................[kW]    (fan motor + recirculating spray pump)
      | water consumption.......[kg]
      | Tnodes.........................[°C]    (inactivity modul)
      | THBout
      mask Help: web(fullfile(path_carnot('help'),'Cooling_Tower.html'),'-helpbrowser')
      mask Display:
      | plot(-20,5,140,80,[20 90 90 20 20],[20 20 70 70 20])
      | plot([30 35],[62 65],[40 35],[62 65],[35 35],[62 65],[80 80],[62 65],[75 80],[62 65],[85 80],[62 65],[57 57],[62 65],[52 57],[62 65],[62 57],[62 65])
      | plot([15 20],[22 22],[15 80],[65 65],[15 15],[22 65],[20 90],[24 24])
      | plot([25 100],[58 58],[25 100],[44 44],[60 25],[51 58],[60 25],[51 44])
      | plot([87 93],[36 36],[87 93],[28 28],[87 82],[36 34],[93 98],[36 34],[87 82],[28 30],[93 98],[28 30],[82 82],[34 30],[98 98],[34 30],[82 95],[34 35],[82 95],[30 29])
      | plot([86 90],[32 32],[90 93],[32 33.5],[90 93],[32 30.5])

== system carnot/Source/Electric_Generator ==
  Inverter : Subsystem  mask(Inverter_simple){P0=9000, ol=1.2, power_steps=[0 0.05 0.1 0.2 0.3 0.5 1 1.2], eta_steps=[0 0.924 0.958 0.974 0.979 0.981 0.98 0.95], standby=0}
      mask prompts: P0 "nominal power"; ol "overload (0.5 ...1.5)"; power_steps "steps for efficiency (0..1..overload)"; eta_steps "efficiency (0..1)"; standby "Standby power consumption in W"
      mask help:
      | This block considers the eficiency of the inverter based on
      | - eta euro [1]
      |
      | In the simple model the efficieny of the inverter is assumed to be constant.
      mask Help: web(fullfile(path_carnot('help'),'Inverter.html'),'-helpbrowser')
      mask Display:
      | %plot([0,0],[0,1],[-0.5,1.5],[0,0],power_steps, eta_steps)
      | plot(-40,0,140,100,[90,10,90,90,10,10],[10,90,90,10,10,90],[40,20],[40,40],[40,20],[30,30],[88,84,75,64,55,50],[70,60,60,80,80,70])
  PV_Generator : Subsystem  mask(PV_Module_simple){Wp=1000, delta_Wp_K=0.0047, fgen=0.91 % 0.06 power missmatch, 0.01 diodes, 0.02 data sheet tolerance}
      mask prompts: Wp "Peak power of the generator [W]"; delta_Wp_K "Temperature coefficient Pmax 1/K"; fgen "efficiency generator field (lossses in diodes, power missmatch, dirt)"
      mask help:
      | This block simultes a pv panel and calculates the output of the module in Ws based on the parameters
      | - Wp of one panel at STC [W]
      | - temperature coefficient of Pmax [1/K]
      | - number of panels [1]
      |
      | Input
      | - weather inclined
      |
      | Output
      | - DC power of the PV generator
      mask Help: web(fullfile(path_carnot('help'),'PV_Generator.html'),'-helpbrowser')
      mask Display: plot(0,0,100,100,[10,40,90,60,10],[10,90,90,10,10],[37,53,60,43,37],[70,70,86,86,70],[60,75,82,67,60],[70,71,86,86,70],[35,30,43,51,35],[65,50,49,65,65],[51,67,73,58,51],[50,50,66,66,50],[28,20,36,43,28],[41,23,23,41,41],[49,44,58,65,49],[41,23,22,41,41])

== system carnot/Source/Energy ==
  Fuel : Subsystem  mask(fuel_source){ft=1, t=20, ls=3.5, p=1.013e5, h_values=[5.14e7 5.69e7], tc=45, price=1, mass=[0.33 0.67 0 0 0 0]}
      mask prompts: ft "fuel (0=no calculation; 1=gaseous; 2=liquid; 3=solid)"; t "temperature [°C]"; ls "stoichiometric air demand [kg/kg]"; p "pressure [Pa]"; h_values "heat without/with condensation [J/kg]"; tc "condensation temperature [°C]"; price "price of fuel per kg [arb. unit]"; mass "massfraction [H C O S N H2O] [-]"
      mask Help: web(fullfile(path_carnot('help'),'Fuel.html'),'-helpbrowser')
  Fuel_CONF : Subsystem  mask(Configurated Condensing Boiler){parameterfile=DefaultFuel_Gas}
      mask prompts: parameterfile "Parameter set"
      mask help:
      | Multinode one-dimensional model of a boiler. Condensing effects are taken in account by an efficiency lookup table.
      | This block uses predefined parameter sets.
      mask init:
      | % path definitions
      | intpath = fullfile(path_carnot('intlibsl'), 'Source','Energy', ...
      |     'Fuel_CONF','parameter_set');
      | pubpath = fullfile(path_carnot('libsl'), 'Source','Energy', ...
      |     'Fuel_CONF','parameter_set');
      | 
      | [namelist, lib] = CarnotCallbacks_getConfNamelist(intpath,pubpath);
      |  
      | if ~lib
      |     myMaskStylesVar{1} = ['popup(', namelist,')'];
      |     set_param(gcb, 'MaskStyles', myMaskStylesVar)
      | end
      | 
      | if exist(fullfile(intpath,[parameterfile '.mat']))
      |     load(fullfile(intpath,parameterfile));
      | else
      |     load(fullfile(pubpath,parameterfile));
      | end
      mask Help: web(fullfile(path_carnot('help'),'Fuel_CONF.html'),'-helpbrowser')
      mask TypeOptions parameterfile: DefaultFuel_Gas

== system carnot/Source/Heat_Exchanger ==
  HeatExchanger : Subsystem  mask(heat exchanger){flowtype=1, ua0=2000, uahot=[0.04 0], uacold=[0.04 0], ualoss=3, cap=10e3, linh=20, quah=10, linc=20, quac=10, t0=20}
      mask prompts: flowtype "type of flow (0 = parallel, 0.5 = cross, 1 = counter)"; ua0 "constant heat transfer ua0 [W/K]"; uahot "[mdot_nom_hot [kg/s] (>0) ,  ua_exp_hot (>=0)]"; uacold "[mdot_nom_cold [kg/s] (>0) ,  ua_exp_cold (>=0)]"; ualoss "heat losses to ambient [W/K]"; cap "capacity [J/K]"; linh "Source: pressure drop linear in massflow [Pa*s/kg]"; quah "Source: pressure drop quadratic in massflow [Pa*s²/kg²]"; linc "Load: pressure drop linear in massflow [Pa*s/kg]"; quac "Load: pressure drop quadratic in massflow [Pa*s²/kg²]"; t0 "initial temperature [degree centigrade]"
      mask help:
      | Calculates the output THV of the hot and cold fluid of a heat exchanger.
      | The heat transfer is:
      | ua = ua0 * ( (mdot_hot/mdot_nom_hot)^ua_exp_hot
      |      + (mdot_cold/mdot_nom_cold)^ua_exp_cold )/2
      mask init:
      | flowtype = max(0, min(flowtype, 1));
      | linh = max(linh,0);
      | linc = max(linc,0);
      | quah = max(quah,0);
      | quac = max(quac,0);
      | uahot(1) = max(uahot(1), 1e-4);
      | uahot(2) = max(uahot(2), 0);
      | uacold(1) = max(uacold(1), 1e-4);
      | uacold(2) = max(uacold(2), 0);
      | cap = max(cap, 0.01);
      mask Help: web(fullfile(path_carnot('help'),'HeatExchanger.html'),'-helpbrowser')
      mask Display:
      | plot(-10,20,115,100,[40,70,70,40,40],[40 40 70 70 40],[55 55 62 48 55 55],[25 40 55 55 70 85],[30 40],[55 55],[70 80],[55 55])
      | port_label('input',1,'Ta')
      | port_label('input',2,'THBpri')
      | port_label('input',3,'THBsec')
      | port_label('output',1,'THBpri')
      | port_label('output',2,'THBsec')
  Radiator : Subsystem  mask(Radiator){pnom=500, dtnom=50, expo=1.3, mcap=5*4182, tini=20, lin=0, qua=1000}
      mask prompts: pnom "nominal power in W"; dtnom "nominal temperature difference in K"; expo "radiator exponent (> 0)"; mcap "mass * capacity per unit in J/K"; tini "initial temperature in degree Celsius"; lin "linear pressure drop dependace of massflow in Pa*s/kg"; qua "quadratic pressure drop dependace of massflow in Pa*s²/kg²"
      mask help:
      | Calculates the power of a radiator according to the nominal power the and the temperature difference (EN 442).
      | Qdot = Qdot_nom * (Tdiff/Tdiff_nom)^n
      | The thermal capacity of the radiator is modeled by a 1-node capacity.
      | mcp*dTnode/dt = mdot*cp*(Tin-Tnode)-Qdot
      | In difference to EN 442 the outlet temperature is Tnode. Tnode is not calculated as average temperature of inlet and outlet.
      | A quadratic pressure drop is applied to the fluid flow.
      mask Help: web(['file:///' fullfile(path_carnot('help'),'Radiator.html')],'-helpbrowser')
      mask Display:
      | plot(-20,0,120,90,[20 90 90 20 20],[20 20 70 70 20],[30 30],[25 65],[40 40],[25 65],[50 50],[25 65],[60 60],[25 65],[70 70],[25 65],[80 80],[25 65],[15 20],[25 25],[15 20],[65 65])
      | port_label('input',1,'Troom')
      | port_label('input',2,'THB')
      | port_label('output',1,'Qdot')
      | port_label('output',2,'THB')
  Radiator_AIV : Subsystem  mask(radiator){pnom=500, dtnom=40, expo=1.3, mcap=5*4182, ra=0.47, tini=20, lin=10, qua=10}
      mask prompts: pnom "nominal power per unit in W"; dtnom "nominal temperature difference in K"; expo "radiator exponent (> 0)"; mcap "mass * capacity per unit in J/K"; ra "radiative part of heat transfer (0..1)"; tini "initial temperature in degree Celsius"; lin "linear pressure drop dependace of massflow in Pa*s/kg"; qua "quadratic pressure drop dependace of massflow in Pa*s²/kg²"
      mask help: Calculates the power of a radiator according to the nominal power the and the temperaure difference.
      mask init:
      | ra = max(0, min(1, ra));
      | co = 1-ra;
      mask Help: web(['file:///' fullfile(path_carnot('help'),'Radiator.html')],'-helpbrowser')
      mask Display:
      | plot(-20,0,120,90,[20 90 90 20 20],[20 20 70 70 20],[30 30],[25 65],[40 40],[25 65],[50 50],[25 65],[60 60],[25 65],[70 70],[25 65],[80 80],[25 65],[15 20],[25 25],[15 20],[65 65])
      | port_label('input',1,'AIV')
      | port_label('input',2,'THB')
      | port_label('output',1,'[S]')
      | port_label('output',2,'THB')
